simulink model "FIR_ref"  (R2020b)
settings: Solver=VariableStepAuto  StartTime=0.0  StopTime=10.0  RelTol=1e-3
settings Model: Creator=Dell  LastModifiedBy=Dell
settings DataIOCC: SaveOutput=off  SaveTime=off

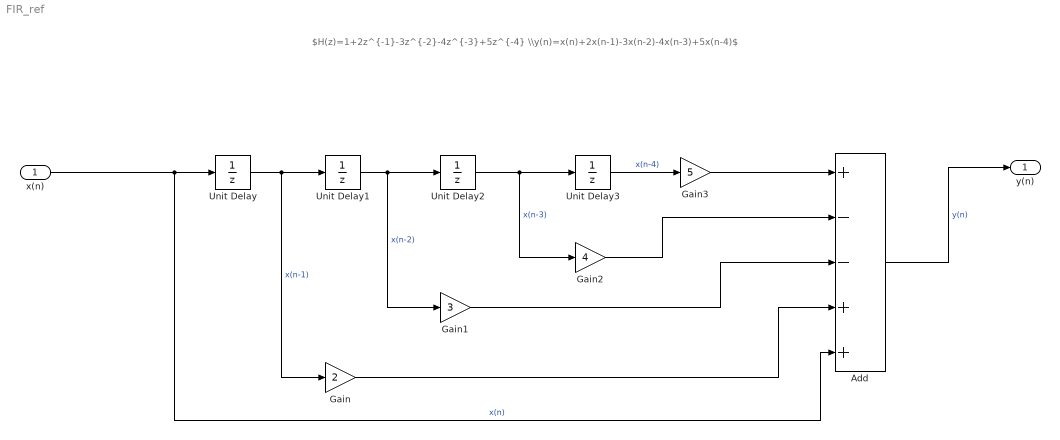
== system FIR_ref ==
  note: $H(z)=1+2z^{-1}-3z^{-2}-4z^{-3}+5z^{-4} \\y(n)=x(n)+2x(n-1)-3x(n-2)-4x(n-3)+5x(n-4)$
  x(n) : Inport  OutDataTypeStr=double  PortDimensions=1  SampleTime=[0,1]
  Add : Sum  Inputs=+--++
  Gain : Gain  Gain=2
  Gain1 : Gain  Gain=3
  Gain2 : Gain  Gain=4
  Gain3 : Gain  Gain=5
  Unit Delay{,1..3} (4 alike) : UnitDelay  InitialCondition=0.1  SampleTime=-1  HasFrameUpgradeWarning=on
  y(n) : Outport  OutDataTypeStr=double  PortDimensions=1  SampleTime=[0,1]
  wires:
  Add/1 -> y(n)/1  "y(n)"
  Gain1/1 -> Add/3
  Unit Delay2/1 -> Unit Delay3/1, Gain2/1  "x(n-3)"
  Unit Delay/1 -> Unit Delay1/1, Gain/1  "x(n-1)"
  Unit Delay3/1 -> Gain3/1  "x(n-4)"
  x(n)/1 -> Unit Delay/1, Add/5  "x(n)"
  Unit Delay1/1 -> Unit Delay2/1, Gain1/1  "x(n-2)"
  Gain2/1 -> Add/2
  Gain/1 -> Add/4
  Gain3/1 -> Add/1
